simulink model "PMSM_Load_Compensation"  (R2019b)
settings: Solver=FixedStepAuto  StartTime=0.0  StopTime=4  FixedStep=2e-5  RelTol=1e-4  EnableMultiTasking=on
InitFcn:
  | Ts = 2e-5
  | Pn = 4
undefined symbols (not defined in the file or in its folder): DiscIntNeverNeededParam
libraries: dsparch4 x8, powerlib x5, simulink x2, powerlib_extras x2, powerlib_meascontrol x1
settings Model: Creator=84360  LastModifiedBy=user
settings DataIOCC: ReturnWorkspaceOutputs=off
settings OptimizationCC: LifeSpan=inf
settings DebuggingCC: SFUnexpectedBacktrackingDiag=warning  SFNoUnconditionalDefaultTransitionDiag=warning  ArithmeticOperatorsInVariantConditions=warning
settings SFSimCC: SimUseLocalCustomCode=off  CustomCodeUndefinedFunction=UseInterfaceOnly
settings RTWCC: RTWUseLocalCustomCode=off
settings CodeAppCC: StateflowObjectComments=on
settings GRTTargetCC: TargetLangStandard=C89/C90 (ANSI)  GeneratePreprocessorConditionals=Disable all
settings ConfigComp: CovMetricSettings=dw  CovHtmlReporting=on  CovSaveCumulativeToWorkspaceVar=on  CovSaveSingleToWorkspaceVar=on  CovExternalEMLEnable=off
settings SimscapeCC: SimscapeNormalizeSystem=off

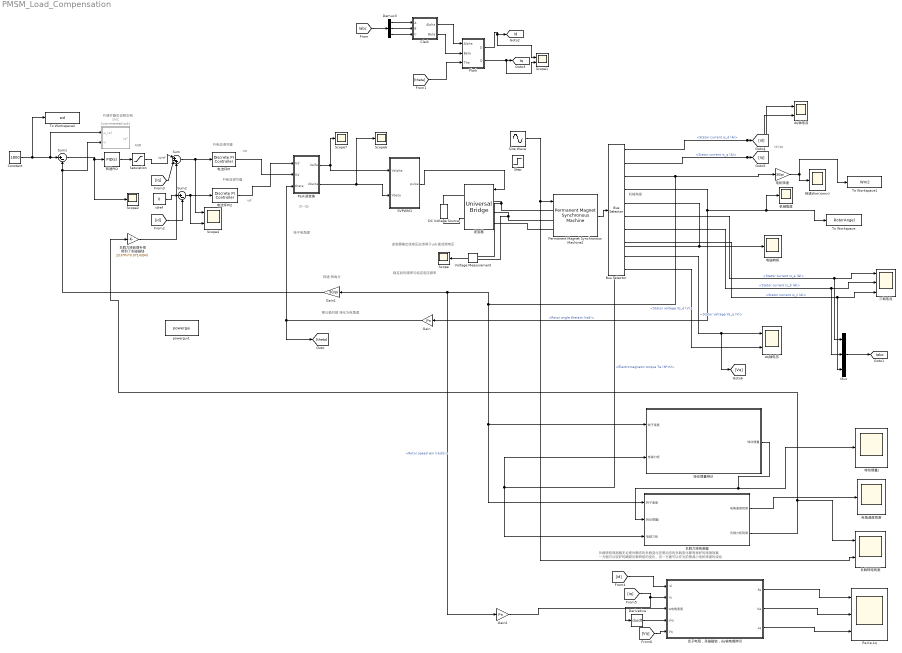
== system PMSM_Load_Compensation ==
  note: 负载转矩观测器无论是对静态的负载变化还是动态的负载变化都有很好的观测效果
      | 一方面可以较好的跟踪负载转矩的变化，另一方面可以作为前馈减小电机转速的波动
  note: PI调节器见说明文档
  note: ASR
  note: 转速 转每分
  note: 转子电角度
  note: 机械角度
  note: 2r--2s
  note: PI电流调节器
  note: ud
  note: uq
  note: iqref
  note: id,iqs
  note: PI电流调节器
  note: 乘以极对数 转化为电角度
  note: 逆变器输出线电压应该等于udc直流测电压
  note: 稳定后的频率与给定电压频率
  Bus Selector : BusSelector  OutputSignals=Stator current is_d (A),Stator current is_q (A),Rotor speed wm (rad/s),Rotor angle thetam (rad),Electromagnetic torque Te (N*m),Stator current is_a (A),Stator current is_b (A),Stator current is_c (A),Stator voltage Vs_q (V),Stator voltage Vs_d (V)
  Clark : Subsystem
  Constant : Constant  Value=1800
  DC Voltage Source : powerlib/Electrical Sources/DC Voltage Source  Amplitude=311  Measurements=None
      settings: SourceProductName=Simscape Electrical
  Demux3 : Demux  Outputs=3
  Derivative : Derivative
  Gain : Gain  Gain=Pn
  Gain1 : Gain  Gain=30/pi
  Gain2 : Gain  Gain=Pn
  Mux : Mux  Inputs=3
  Park逆变换 : Subsystem
  Permanent Magnet Synchronous Machine2 : powerlib/Machines/Permanent Magnet Synchronous Machine  NbPhases=3  FluxDistribution=Sinusoidal  RotorType=Round  MechanicalLoad=Torque Tm  PresetModel=No  ShowDetailedParameters=on  MeasurementBus=off  Resistance=0.18  Inductance=8.5e-3  dqInductances=[0.00309 0.00309]  La=0.000835  MachineConstant=Flux linkage established by magnets (V.s)  Flux=0.0714394  VoltageCst=51.8307  TorqueCst=0.42864  Flat=120  Mechanical=[0.000621417 0.000303448 4]  PolePairs=4  InitialConditions=[0,0, 0,0]  InitialConditions5ph=[0 0 0 0 0 0]  RefAngle=Aligned with phase A axis (original Park)  IterativeDiscreteModel=Trapezoidal non iterative  TsBlock=-1  TsPowergui=0
  Plark : Subsystem
  Rs,Ke,Lq : Scope  NumInputPorts=3
  SMC : Subsystem  Commented=on
  SVPWM1 : Subsystem
  Saturation : Saturate  UpperLimit=50  LowerLimit=-50
  Scope{,2,6..7} (4 alike) : Scope
  Scope1 : Scope  NumInputPorts=2
  Scope4 : Scope  NumInputPorts=2
  Sine Wave : Sin  Amplitude=15  Frequency=2  SampleTime=0
  Step : Step  Before=5  After=10  SampleTime=0
  Sum : Sum  Inputs=|+-+
  Sum1 : Sum  Inputs=|+-
  Sum2 : Sum  Inputs=|+-
  To Workspace : ToWorkspace  VariableName=RotorAngel  SaveFormat=Timeseries  SampleTime=-1
  To Workspace1 : ToWorkspace  VariableName=Wm2  SaveFormat=Timeseries  SampleTime=-1
  To Workspace2 : ToWorkspace  VariableName=wd  SaveFormat=Timeseries  SampleTime=-1
  Voltage Measurement : powerlib/Measurements/Voltage Measurement  PhasorSimulation=off  OutputType=Complex  PSBequivalent=0
      settings: SourceProductName=Simscape Electrical
  dq轴电压 : Scope  NumInputPorts=2
  dq轴电流 : Scope  NumInputPorts=2
  idref : Constant  Value=0
  powergui1 : powerlib/powergui  SimulationMode=Discrete  SampleTime=2e-5  frequency=60  Iterations=50  frequencyindice=0  Pbase=100e6  ErrMax=1e-4  UnitsV=kV  UnitsW=MW  buscounter=0  FunctionMessages=off  echomessages=off  EnableUseOfTLC=off  CurrentSourceSwitches=off  DisableSnubberDevices=off  DisableRonSwitches=off  DisableVfSwitches=off  DisplayEquations=off  AutomaticDiscreteSolvers=off  SolverType=Tustin/Backward Euler (TBE)  Interpol=off  ExternalGateDelay=off  methode=off  Ts=100  x0status=blocks  SPID=off  SwTol=0  HookPort=off  NonlinearTolerance=1e-4  nMaxIteration=100  ContinueOnMaxIteration=off  RestoreLinks=warning  ResistiveCurrentMeasurement=off  Frange=[0:2:500]  Ylog=off  Xlog=on  ShowGrid=off  save=off  variable=ZData  structure=0  ZoomFFT=on  StartTime=0.0  cycles=1  DisplayStyle=1  fundamental=60  FreqAxis=off  MaxFrequency=1000  frequencyindicesteady=1  RmsSteady=1  display=off
      settings: SourceProductName=Simscape Electrical
  三相电流 : Scope  NumInputPorts=3
  定子电阻，永磁磁链，dq轴电感辨识 : Subsystem
  机械角度 : Scope
  电机转速 : Gain  Gain=30/pi
  电流环PI : powerlib_extras/Discrete  Control Blocks/Discrete PI Controller  Kp=8.5e-3*2100  Ki=2.875*2100  Par_Limits=[250 -250]  Init=0  Ts=Ts
      settings: SourceProductName=Simscape Electrical
  电流环PI2 : powerlib_extras/Discrete  Control Blocks/Discrete PI Controller  Kp=8.5e-3*2100  Ki=2.875*2100  Par_Limits=[250 -250]  Init=0  Ts=Ts
      settings: SourceProductName=Simscape Electrical
  电磁转矩 : Scope
  电角速度观测 : Scope
  负载力矩前馈补偿 用到了永磁磁链 : Gain  Gain=2/(3*Pn*0.0714394)
  负载力矩观测器 : Subsystem
  负载转矩观测 : Scope  NumInputPorts=2
  转动惯量J : Scope
  转动惯量辨识 : Subsystem
  转速PID : simulink/Continuous/PID Controller  Controller=PID  Form=Parallel  TimeDomain=Continuous-time  SampleTime=-1  IntegratorMethod=Forward Euler  FilterMethod=Forward Euler  ControllerParametersSource=internal  P=0.476  I=2.3810  D=0  UseFilter=on  N=100  TunerSelectOption=Transfer Function Based (PID Tuner App)  InitialConditionSource=internal  InitialConditionForIntegrator=0  InitialConditionForFilter=0  DifferentiatorICPrevScaledInput=0  ExternalReset=none  TrackingMode=off  Kt=1  LimitOutput=off  UpperSaturationLimit=inf  LowerSaturationLimit=-inf  LinearizeAsGain=on  AntiWindupMode=none  Kb=1  POutMin=[]  POutMax=[]  IOutMin=[]  IOutMax=[]  DOutMin=[]  DOutMax=[]  NOutMin=[]  NOutMax=[]  SumOutMin=[]  SumOutMax=[]  SaturationOutMin=[]  SaturationOutMax=[]  PParamMin=[]  PParamMax=[]  IParamMin=[]  IParamMax=[]  DParamMin=[]  DParamMax=[]  NParamMin=[]  NParamMax=[]  KbParamMin=[]  KbParamMax=[]  KtParamMin=[]  KtParamMax=[]  KbOutMin=[]  KbOutMax=[]  KtOutMin=[]  KtOutMax=[]  IntegratorOutMin=[]  IntegratorOutMax=[]  FilterOutMin=[]  FilterOutMax=[]  SumI1OutMin=[]  SumI1OutMax=[]  SumI2OutMin=[]  SumI2OutMax=[]  SumI3OutMin=[]  SumI3OutMax=[]  SumI4OutMin=[]  SumI4OutMax=[]  SumDOutMin=[]  SumDOutMax=[]  DifferentiatorOutMin=[]  DifferentiatorOutMax=[]  FilterDiffOutCoefMin=[]  FilterDiffOutCoefMax=[]  ReciprocalOutMin=[]  ReciprocalOutMax=[]  SumDenOutMin=[]  SumDenOutMax=[]  SumNumOutMin=[]  SumNumOutMax=[]  DivideOutMin=[]  DivideOutMax=[]  IntegratorContinuousStateAttributes=''  IntegratorStateMustResolveToSignalObject=off  IntegratorRTWStateStorageClass=Auto  FilterContinuousStateAttributes=''  FilterStateMustResolveToSignalObject=off  FilterRTWStateStorageClass=Auto  ParallelPVariant=InternalParameters  IdealPVariant=Disabled  IVariant=InternalParameters  DVariant=InternalParameters  IntegratorVariant=Continuous  SatVariant=Disabled  AWVariant=Passthrough  PCopyVariant=Disabled  TRVariant=Disabled  FdbkBlocksVariant=Forward  IdealPFdbkVariant=Disabled  SatFdbkVariant=Disabled  DerivativeFilterVariant=ContFilter  NVariant=InternalParameters  NCopyVariant=Disabled  FilterICVariant=InternalICsFilter  IntegratorICVariant=InternalICs  ExternalResetVariant=Disabled  TRSumVariant=Passthrough  SumFdbkVariant=Disabled  SumVariant=Sum_PID
  转速Wm(r/min) : Scope
  逆变器 : powerlib/Power Electronics/Universal Bridge  Arms=3  SnubberResistance=1e5  SnubberCapacitance=inf  Device=IGBT / Diodes  Ron=1e-3  Lon=0  ForwardVoltages="[  0  0  ]"  ForwardVoltage=0  GTOparameters=[ 10e-6 , 20e-6 ]  IGBTparameters=[ 1e-6 , 2e-6 ]  Measurements=All voltages and currents  Measurements_2=None  converterType=Rectifier
      settings: SourceProductName=Simscape Electrical
  tag scope: Iabc=global, Id=global, Iq=global
  wires:
  Park逆变换/1(Ualfa) -> SVPWM1/1(Valpha), Scope7/1
  SVPWM1/1(pulse) -> 逆变器/1
  Voltage Measurement/1 -> Scope/1
  电流环PI/1 -> Park逆变换/2(Uq')
  Sum2/1 -> Scope4/2, 电流环PI2/1
  电流环PI2/1 -> Park逆变换/1(Ud')
  Permanent Magnet Synchronous Machine2/1 -> Bus Selector/1
  idref/1 -> Sum2/1
  Sum1/1 -> Scope2/1, 转速PID/1
  Bus Selector/4 -> To Workspace/1, 机械角度/1, Gain/1  "<Rotor angle thetam (rad)>"
  Bus Selector/3 -> 电机转速/1, Gain2/1, Gain1/1, 负载力矩观测器/1(转子速度), 转动惯量辨识/1(转子速度)  "<Rotor speed wm (rad/s)>"
  Gain/1 -> [theta], Park逆变换/3(theta)
  Bus Selector/6 -> Mux/1, 三相电流/1  "<Stator current is_a (A)>"
  Bus Selector/7 -> Mux/2, 三相电流/2  "<Stator current is_b (A)>"
  Bus Selector/8 -> Mux/3, 三相电流/3  "<Stator current is_c (A)>"
  Park逆变换/2(Ubeita) -> SVPWM1/2(Vbeta), Scope6/1
  Gain1/1 -> SMC/2(w), Sum1/2
  电机转速/1 -> To Workspace1/1, 转速Wm(r/min)/1
  Mux/1 -> [Iabc]
  [Iabc] -> Demux3/1
  Demux3/2 -> Clark/2(B)
  Plark/2(Q) -> Scope1/2, [Iq]
  Demux3/3 -> Clark/3(C)
  Clark/2(Beta) -> Plark/2(Beta)
  Demux3/1 -> Clark/1(A)
  Clark/1(Alpha) -> Plark/1(Alpha)
  [theta] -> Plark/3(The)
  Plark/1(D) -> Scope1/1, [Id]
  Saturation/1 -> Sum/1
  [iq] -> Sum/2
  [id] -> Sum2/2
  Bus Selector/9 -> [Vq], dq轴电压/1  "<Stator voltage Vs_q (V)>"
  Constant/1 -> To Workspace2/1, SMC/1(w_ref), Sum1/1
  Sum/1 -> Scope4/1, 电流环PI/1
  转速PID/1 -> Saturation/1
  Bus Selector/5 -> 电磁转矩/1, 负载力矩观测器/3(电磁力矩), 转动惯量辨识/2(电磁力矩)  "<Electromagnetic torque Te (N*m)>"
  负载力矩观测器/1(电角速度观测) -> 电角速度观测/1
  负载力矩观测器/2(负载力矩观测) -> 负载转矩观测/1, 负载力矩前馈补偿 用到了永磁磁链/1
  Sine Wave/1 -> 负载转矩观测/2, Permanent Magnet Synchronous Machine2/1
  转动惯量辨识/1(转动惯量) -> 负载力矩观测器/2(转动惯量J), 转动惯量J/1
  Bus Selector/1 -> dq轴电流/1, [id]  "<Stator current is_d (A)>"
  Bus Selector/10 -> dq轴电压/2  "<Stator voltage Vs_d (V)>"
  Bus Selector/2 -> dq轴电流/2, [iq]  "<Stator current is_q (A)>"
  负载力矩前馈补偿 用到了永磁磁链/1 -> Sum/3
  定子电阻，永磁磁链，dq轴电感辨识/1(Rs) -> Rs,Ke,Lq/1
  定子电阻，永磁磁链，dq轴电感辨识/2(Ke) -> Rs,Ke,Lq/2
  定子电阻，永磁磁链，dq轴电感辨识/3(Lq) -> Rs,Ke,Lq/3
  [id] -> 定子电阻，永磁磁链，dq轴电感辨识/1(id)
  [iq] -> Derivative/1, 定子电阻，永磁磁链，dq轴电感辨识/2(iq)
  Derivative/1 -> 定子电阻，永磁磁链，dq轴电感辨识/4(diq)
  Gain2/1 -> 定子电阻，永磁磁链，dq轴电感辨识/3(w电角速度)
  [Vq] -> 定子电阻，永磁磁链，dq轴电感辨识/5(Vq)
  connections:
  Voltage Measurement/LConn1 -- Permanent Magnet Synchronous Machine2/LConn1 -- 逆变器/LConn1
  Voltage Measurement/LConn2 -- 逆变器/LConn2 -- Permanent Magnet Synchronous Machine2/LConn2
  DC Voltage Source/RConn1 -- 逆变器/RConn1
  DC Voltage Source/LConn1 -- 逆变器/RConn2
  Permanent Magnet Synchronous Machine2/LConn3 -- 逆变器/LConn3

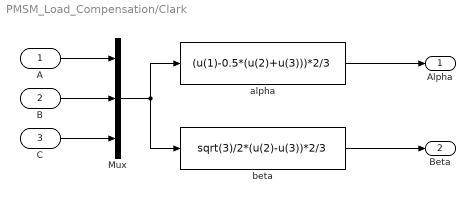
== system PMSM_Load_Compensation/Clark ==
  A : Inport
  B : Inport  Port=2
  C : Inport  Port=3
  Mux : Mux  Inputs=3
  alpha : Fcn  Expr=(u(1)-0.5*(u(2)+u(3)))*2/3
  beta : Fcn  Expr=sqrt(3)/2*(u(2)-u(3))*2/3
  Alpha : Outport
  Beta : Outport  Port=2
  wires:
  alpha/1 -> Alpha/1
  B/1 -> Mux/2
  C/1 -> Mux/3
  A/1 -> Mux/1
  Mux/1 -> beta/1, alpha/1
  beta/1 -> Beta/1

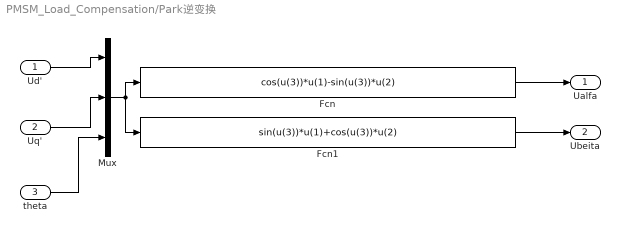
== system PMSM_Load_Compensation/Park逆变换 ==
  Ud' : Inport
  Uq' : Inport  Port=2
  theta : Inport  Port=3
  Fcn : Fcn  Expr=cos(u(3))*u(1)-sin(u(3))*u(2)
  Fcn1 : Fcn  Expr=sin(u(3))*u(1)+cos(u(3))*u(2)
  Mux : Mux  Inputs=3
  Ualfa : Outport
  Ubeita : Outport  Port=2
  wires:
  Mux/1 -> Fcn1/1, Fcn/1
  Fcn1/1 -> Ubeita/1
  Uq'/1 -> Mux/2
  Ud'/1 -> Mux/1
  Fcn/1 -> Ualfa/1
  theta/1 -> Mux/3

== system PMSM_Load_Compensation/Plark ==
  Alpha : Inport
  Beta : Inport  Port=2
  The : Inport  Port=3
  Mux : Mux  Inputs=3
  d : Fcn  Expr=u(1)*cos(u(3))+u(2)*sin(u(3))
  q : Fcn  Expr=-u(1)*sin(u(3))+u(2)*cos(u(3))
  D : Outport
  Q : Outport  Port=2
  wires:
  d/1 -> D/1
  Beta/1 -> Mux/2
  Alpha/1 -> Mux/1
  Mux/1 -> q/1, d/1
  q/1 -> Q/1
  The/1 -> Mux/3

== system PMSM_Load_Compensation/SMC ==
  w_ref : Inport
  w : Inport  Port=2
  Discrete-Time Integrator : DiscreteIntegrator  SampleTime=-1  ICPrevOutput=DiscIntNeverNeededParam  ICPrevScaledInput=DiscIntNeverNeededParam
  Mux1 : Mux  Inputs=3
  S-Function : S-Function  FunctionName=FOC_SMC  SFunctionDeploymentMode=off  EnableBusSupport=off
  Sum4 : Sum  Inputs=|+-
  iq* : Outport
  wires:
  w/1 -> Sum4/2, Mux1/2
  Sum4/1 -> Discrete-Time Integrator/1
  w_ref/1 -> Sum4/1, Mux1/1
  Discrete-Time Integrator/1 -> Mux1/3
  Mux1/1 -> S-Function/1
  S-Function/1 -> iq*/1

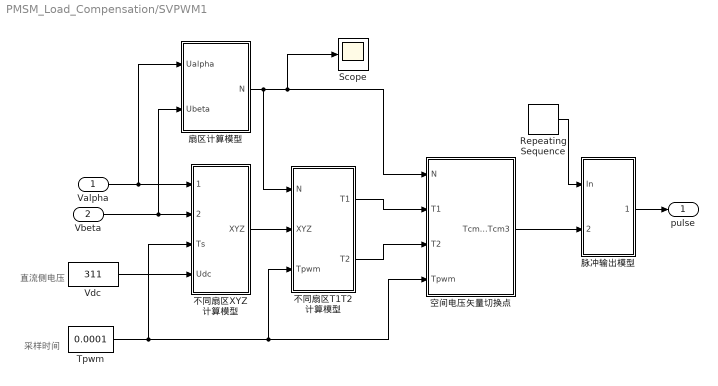
== system PMSM_Load_Compensation/SVPWM1 ==
  note: 采样时间
  note: 直流侧电压
  Valpha : Inport
  Vbeta : Inport  Port=2
  Repeating Sequence : simulink/Sources/Repeating Sequence  rep_seq_t=[0 0.00005 0.0001]  rep_seq_y=[0 0.00005 0]
  Scope : Scope
  Tpwm : Constant  Value=0.0001
  Vdc : Constant  Value=311
  不同扇区T1T2 计算模型 : Subsystem
  不同扇区XYZ 计算模型 : Subsystem
  扇区计算模型 : Subsystem
  空间电压矢量切换点 : Subsystem
  脉冲输出模型 : Subsystem
  pulse : Outport
  wires:
  脉冲输出模型/1(PWM) -> pulse/1
  Repeating Sequence/1 -> 脉冲输出模型/1(In)
  Vbeta/1 -> 不同扇区XYZ 计算模型/2(Ubeta), 扇区计算模型/2(Ubeta)
  不同扇区T1T2 计算模型/1(T1) -> 空间电压矢量切换点/2(T1)
  Valpha/1 -> 不同扇区XYZ 计算模型/1(Ualpha), 扇区计算模型/1(Ualpha)
  不同扇区T1T2 计算模型/2(T2) -> 空间电压矢量切换点/3(T2)
  扇区计算模型/1("N ") -> Scope/1, 空间电压矢量切换点/1(N), 不同扇区T1T2 计算模型/1(N)
  不同扇区XYZ 计算模型/1(XYZ) -> 不同扇区T1T2 计算模型/2(XYZ)
  Tpwm/1 -> 不同扇区XYZ 计算模型/3(Ts), 空间电压矢量切换点/4(Tpwm), 不同扇区T1T2 计算模型/3(Tpwm)
  Vdc/1 -> 不同扇区XYZ 计算模型/4(Udc)
  空间电压矢量切换点/1(Tcm1 Tcm2 Tcm3) -> 脉冲输出模型/2(Tcm123)

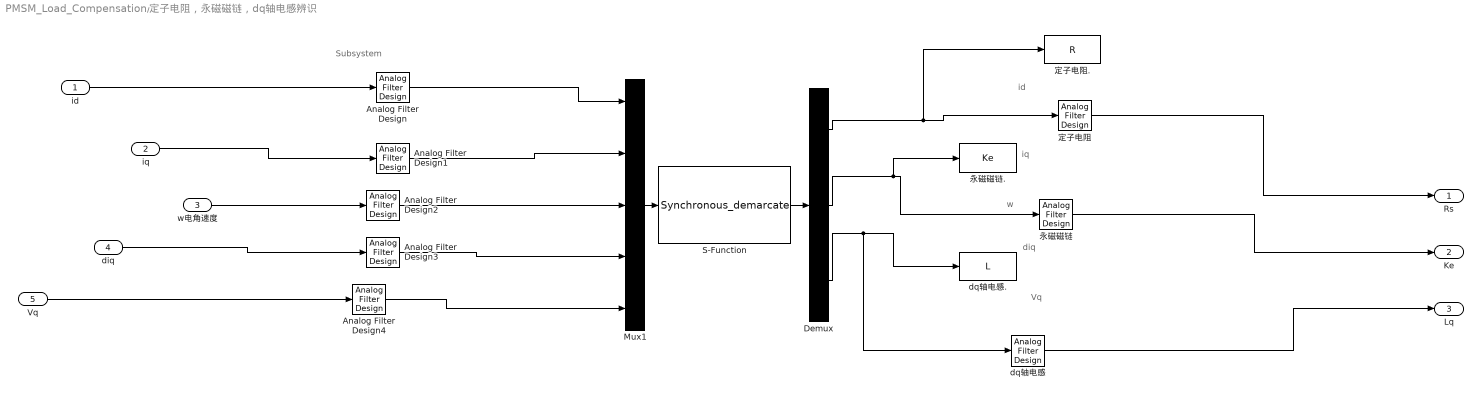
== system PMSM_Load_Compensation/定子电阻，永磁磁链，dq轴电感辨识 ==
  note: Subsystem
  note: id
  note: iq
  note: w
  note: diq
  note: Vq
  id : Inport
  iq : Inport  Port=2
  w电角速度 : Inport  Port=3
  diq : Inport  Port=4
  Vq : Inport  Port=5
  Analog Filter Design{,1..4} (5 alike) : dsparch4/Analog Filter Design  method=Butterworth  filttype=Lowpass  N=8  Wlo=50  Whi=80  Rp=2  Rs=40
  Demux : Demux  Outputs=3
  Mux1 : Mux  Inputs=5
  S-Function : S-Function  FunctionName=Synchronous_demarcate  SFunctionDeploymentMode=off  EnableBusSupport=off
  dq轴电感 : dsparch4/Analog Filter Design  method=Butterworth  filttype=Lowpass  N=8  Wlo=20  Whi=80  Rp=2  Rs=40
  dq轴电感. : ToWorkspace  VariableName=L  SaveFormat=Timeseries  SampleTime=-1
  定子电阻 : dsparch4/Analog Filter Design  method=Butterworth  filttype=Lowpass  N=8  Wlo=20  Whi=80  Rp=2  Rs=40
  定子电阻. : ToWorkspace  VariableName=R  SaveFormat=Timeseries  SampleTime=-1
  永磁磁链 : dsparch4/Analog Filter Design  method=Butterworth  filttype=Lowpass  N=8  Wlo=20  Whi=80  Rp=2  Rs=40
  永磁磁链. : ToWorkspace  VariableName=Ke  SaveFormat=Timeseries  SampleTime=-1
  Rs : Outport
  Ke : Outport  Port=2
  Lq : Outport  Port=3
  wires:
  diq/1 -> Analog Filter Design3/1
  永磁磁链/1 -> Ke/1
  iq/1 -> Analog Filter Design1/1
  定子电阻/1 -> Rs/1
  w电角速度/1 -> Analog Filter Design2/1
  S-Function/1 -> Demux/1
  id/1 -> Analog Filter Design/1
  Demux/2 -> 永磁磁链./1, 永磁磁链/1
  Analog Filter Design3/1 -> Mux1/4
  Demux/1 -> 定子电阻./1, 定子电阻/1
  Mux1/1 -> S-Function/1
  Vq/1 -> Analog Filter Design4/1
  Analog Filter Design2/1 -> Mux1/3
  dq轴电感/1 -> Lq/1
  Demux/3 -> dq轴电感./1, dq轴电感/1
  Analog Filter Design4/1 -> Mux1/5
  Analog Filter Design/1 -> Mux1/1
  Analog Filter Design1/1 -> Mux1/2

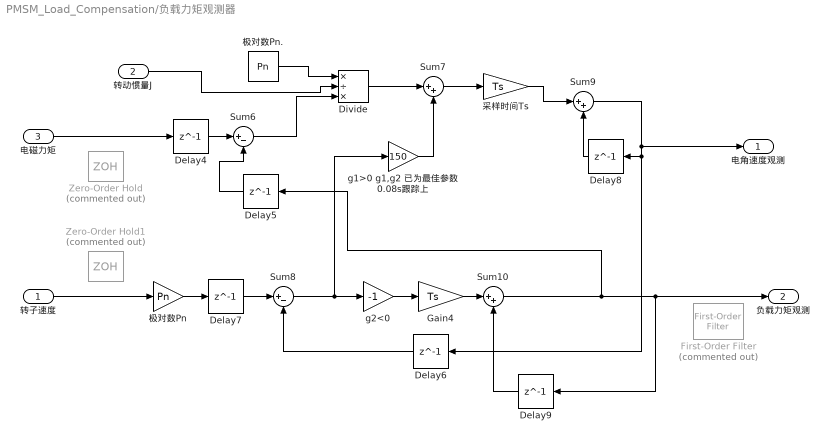
== system PMSM_Load_Compensation/负载力矩观测器 ==
  转子速度 : Inport
  转动惯量J : Inport  Port=2
  电磁力矩 : Inport  Port=3
  Delay{4..9} (6 alike) : Delay  DelayLength=1  InitialCondition=0
  Divide : Product  Inputs=*/*
  First-Order Filter : powerlib_meascontrol/Filters/First-Order Filter  Commented=on  FilterType=Lowpass  Tc=10e-3  Ts=0  Initialize=on  Vac_Init=[0, 0, 200]  Vdc_Init=0  PlotResponse=off  FreqRange="[0,  200,  1]"
      settings: SourceProductName=Simscape Electrical
  Gain4 : Gain  Gain=Ts
  Sum10 : Sum  Inputs=|++
  Sum6 : Sum  Inputs=|+-
  Sum7 : Sum  Inputs=|++
  Sum8 : Sum  Inputs=|+-
  Sum9 : Sum  Inputs=|++
  Zero-Order Hold : ZeroOrderHold  Commented=on  SampleTime=-1
  Zero-Order Hold1 : ZeroOrderHold  Commented=on  SampleTime=-1
  g1>0 g1,g2 已为最佳参数 0.08s跟踪上 : Gain  Gain=150
  g2<0 : Gain  Gain=-1
  极对数Pn : Gain  Gain=Pn
  极对数Pn. : Constant  Value=Pn
  采样时间Ts : Gain  Gain=Ts
  电角速度观测 : Outport
  负载力矩观测 : Outport  Port=2
  wires:
  Sum9/1 -> 电角速度观测/1, Delay8/1, Delay6/1
  Sum6/1 -> Divide/3
  极对数Pn/1 -> Delay7/1
  Sum7/1 -> 采样时间Ts/1
  Delay6/1 -> Sum8/2
  Delay5/1 -> Sum6/2
  g1>0 g1,g2 已为最佳参数 0.08s跟踪上/1 -> Sum7/2
  Sum8/1 -> g1>0 g1,g2 已为最佳参数 0.08s跟踪上/1, g2<0/1
  Delay7/1 -> Sum8/1
  采样时间Ts/1 -> Sum9/1
  Gain4/1 -> Sum10/1
  Delay8/1 -> Sum9/2
  Divide/1 -> Sum7/1
  g2<0/1 -> Gain4/1
  Delay9/1 -> Sum10/2
  极对数Pn./1 -> Divide/1
  Delay4/1 -> Sum6/1
  转动惯量J/1 -> Divide/2
  Sum10/1 -> Delay5/1, 负载力矩观测/1, Delay9/1
  电磁力矩/1 -> Delay4/1
  转子速度/1 -> 极对数Pn/1

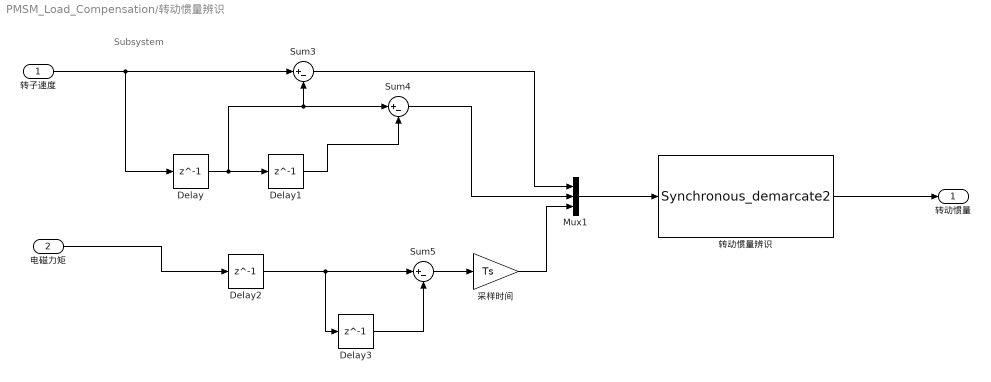
== system PMSM_Load_Compensation/转动惯量辨识 ==
  note: Subsystem
  转子速度 : Inport
  电磁力矩 : Inport  Port=2
  Delay{,1..3} (4 alike) : Delay  DelayLength=1  InitialCondition=0
  Mux1 : Mux  Inputs=3
  Sum3 : Sum  Inputs=|+-
  Sum4 : Sum  Inputs=|+-
  Sum5 : Sum  Inputs=|+-
  转动惯量辨识 : S-Function  FunctionName=Synchronous_demarcate2  SFunctionDeploymentMode=off  EnableBusSupport=off
  采样时间 : Gain  Gain=Ts
  转动惯量 : Outport
  wires:
  Mux1/1 -> 转动惯量辨识/1
  Sum5/1 -> 采样时间/1
  Delay1/1 -> Sum4/2
  采样时间/1 -> Mux1/3
  Delay/1 -> Sum3/2, Sum4/1, Delay1/1
  Sum3/1 -> Mux1/1
  Sum4/1 -> Mux1/2
  转子速度/1 -> Delay/1, Sum3/1
  Delay3/1 -> Sum5/2
  Delay2/1 -> Delay3/1, Sum5/1
  电磁力矩/1 -> Delay2/1
  转动惯量辨识/1 -> 转动惯量/1

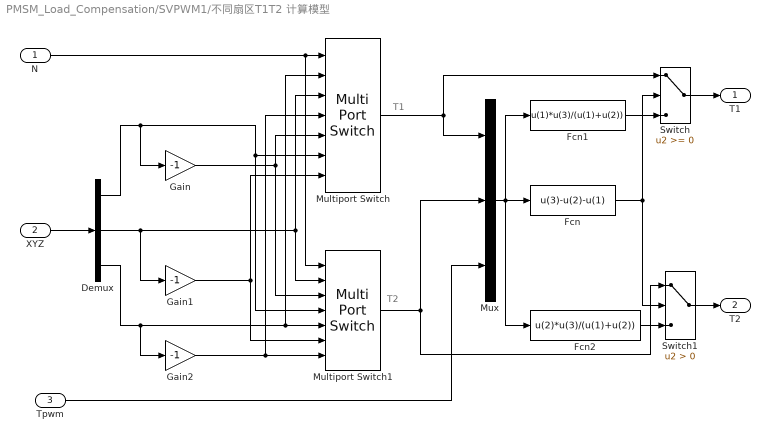
== system PMSM_Load_Compensation/SVPWM1/不同扇区T1T2 计算模型 ==
  note: T1
  note: T2
  N : Inport
  XYZ : Inport  Port=2
  Tpwm : Inport  Port=3
  Demux : Demux  Outputs=3
  Fcn : Fcn  Expr=u(3)-u(2)-u(1)
  Fcn1 : Fcn  Expr=u(1)*u(3)/(u(1)+u(2))
  Fcn2 : Fcn  Expr=u(2)*u(3)/(u(1)+u(2))
  Gain : Gain  Gain=-1
  Gain1 : Gain  Gain=-1
  Gain2 : Gain  Gain=-1
  Multiport Switch : MultiPortSwitch  Inputs=6  DiagnosticForDefault=Warning
  Multiport Switch1 : MultiPortSwitch  Inputs=6  DiagnosticForDefault=Warning
  Mux : Mux  Inputs=3
  Switch : Switch
  Switch1 : Switch  Criteria=u2 > Threshold
  T1 : Outport
  T2 : Outport  Port=2
  wires:
  Tpwm/1 -> Mux/3
  XYZ/1 -> Demux/1
  Switch1/1 -> T2/1
  Switch/1 -> T1/1
  Fcn2/1 -> Switch1/3
  Fcn1/1 -> Switch/3
  Fcn/1 -> Switch/2, Switch1/2
  Mux/1 -> Fcn1/1, Fcn/1, Fcn2/1
  Multiport Switch/1 -> Switch/1, Mux/1
  Multiport Switch1/1 -> Switch1/1, Mux/2
  N/1 -> Multiport Switch/1, Multiport Switch1/1
  Demux/2 -> Multiport Switch/3, Multiport Switch1/2, Gain1/1
  Demux/3 -> Multiport Switch1/5, Multiport Switch/2, Gain2/1
  Demux/1 -> Multiport Switch/6, Multiport Switch1/4, Gain/1
  Gain/1 -> Multiport Switch1/3, Multiport Switch/5
  Gain2/1 -> Multiport Switch/4, Multiport Switch1/7
  Gain1/1 -> Multiport Switch1/6, Multiport Switch/7

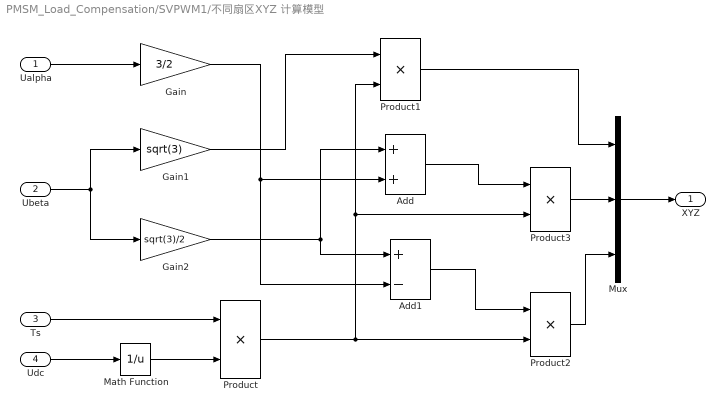
== system PMSM_Load_Compensation/SVPWM1/不同扇区XYZ 计算模型 ==
  Ualpha : Inport
  Ubeta : Inport  Port=2
  Ts : Inport  Port=3
  Udc : Inport  Port=4
  Add : Sum
  Add1 : Sum  Inputs=+-
  Gain : Gain  Gain=3/2
  Gain1 : Gain  Gain=sqrt(3)
  Gain2 : Gain  Gain=sqrt(3)/2
  Math Function : Math  Operator=reciprocal  SaturateOnIntegerOverflow=on
  Mux : Mux  Inputs=3
  Product{,1..3} (4 alike) : Product  RndMeth=Zero
  XYZ : Outport
  wires:
  Mux/1 -> XYZ/1
  Product1/1 -> Mux/1
  Product3/1 -> Mux/2
  Product2/1 -> Mux/3
  Ualpha/1 -> Gain/1
  Ubeta/1 -> Gain2/1, Gain1/1
  Udc/1 -> Math Function/1
  Math Function/1 -> Product/2
  Ts/1 -> Product/1
  Gain1/1 -> Product1/1
  Product/1 -> Product2/2, Product1/2, Product3/2
  Gain/1 -> Add1/2, Add/2
  Gain2/1 -> Add/1, Add1/1
  Add1/1 -> Product2/1
  Add/1 -> Product3/1

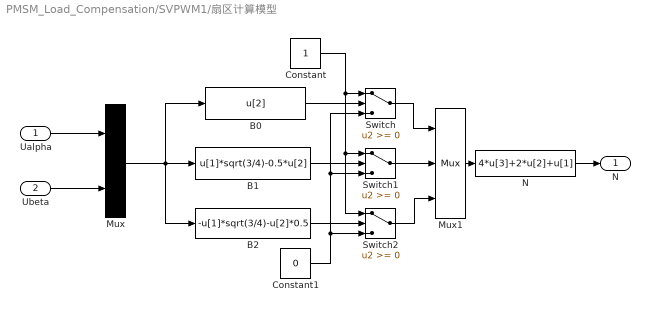
== system PMSM_Load_Compensation/SVPWM1/扇区计算模型 ==
  Ualpha : Inport
  Ubeta : Inport  Port=2
  B0 : Fcn  Expr=u[2]
  B1 : Fcn  Expr=u[1]*sqrt(3/4)-0.5*u[2]
  B2 : Fcn  Expr=-u[1]*sqrt(3/4)-u[2]*0.5
  Constant : Constant
  Constant1 : Constant  Value=0
  Mux : Mux  Inputs=2
  Mux1 : Mux  Inputs=3
  N : Fcn  Expr=4*u[3]+2*u[2]+u[1]
  Switch : Switch
  Switch1 : Switch
  Switch2 : Switch
  "N " : Outport
  wires:
  Switch2/1 -> Mux1/3
  Switch/1 -> Mux1/1
  Ualpha/1 -> Mux/1
  Ubeta/1 -> Mux/2
  Mux/1 -> B2/1, B1/1, B0/1
  B0/1 -> Switch/2
  B1/1 -> Switch1/2
  B2/1 -> Switch2/2
  Constant/1 -> Switch/1, Switch2/1, Switch1/1
  Constant1/1 -> Switch/3, Switch1/3, Switch2/3
  Switch1/1 -> Mux1/2
  Mux1/1 -> N/1
  N/1 -> "N "/1

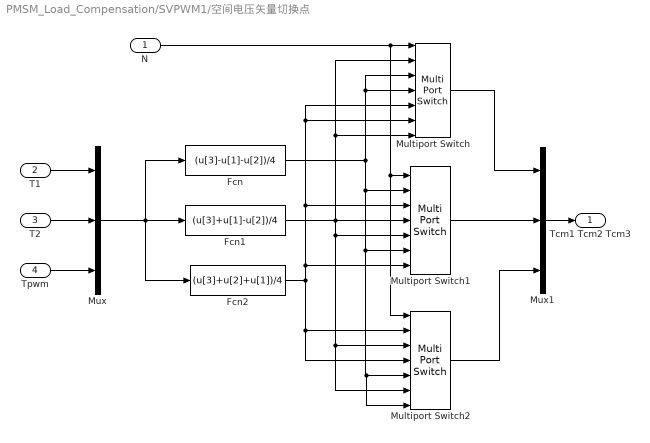
== system PMSM_Load_Compensation/SVPWM1/空间电压矢量切换点 ==
  N : Inport
  T1 : Inport  Port=2
  T2 : Inport  Port=3
  Tpwm : Inport  Port=4
  Fcn : Fcn  Expr=(u[3]-u[1]-u[2])/4
  Fcn1 : Fcn  Expr=(u[3]+u[1]-u[2])/4
  Fcn2 : Fcn  Expr=(u[3]+u[2]+u[1])/4
  Multiport Switch : MultiPortSwitch  Inputs=6  DiagnosticForDefault=Warning
  Multiport Switch1 : MultiPortSwitch  Inputs=6  DiagnosticForDefault=Warning
  Multiport Switch2 : MultiPortSwitch  Inputs=6  DiagnosticForDefault=Warning
  Mux : Mux  Inputs=3
  Mux1 : Mux  Inputs=3
  Tcm1 Tcm2 Tcm3 : Outport
  wires:
  Mux/1 -> Fcn2/1, Fcn/1, Fcn1/1
  Tpwm/1 -> Mux/3
  T2/1 -> Mux/2
  T1/1 -> Mux/1
  Multiport Switch2/1 -> Mux1/3
  Multiport Switch1/1 -> Mux1/2
  Multiport Switch/1 -> Mux1/1
  Mux1/1 -> Tcm1 Tcm2 Tcm3/1
  Fcn/1 -> Multiport Switch/3, Multiport Switch/4, Multiport Switch1/6, Multiport Switch2/5, Multiport Switch2/7, Multiport Switch1/2
  Fcn1/1 -> Multiport Switch1/5, Multiport Switch2/3, Multiport Switch2/6, Multiport Switch1/4, Multiport Switch/7, Multiport Switch/2
  Fcn2/1 -> Multiport Switch/5, Multiport Switch/6, Multiport Switch1/3, Multiport Switch1/7, Multiport Switch2/2, Multiport Switch2/4
  N/1 -> Multiport Switch2/1, Multiport Switch1/1, Multiport Switch/1

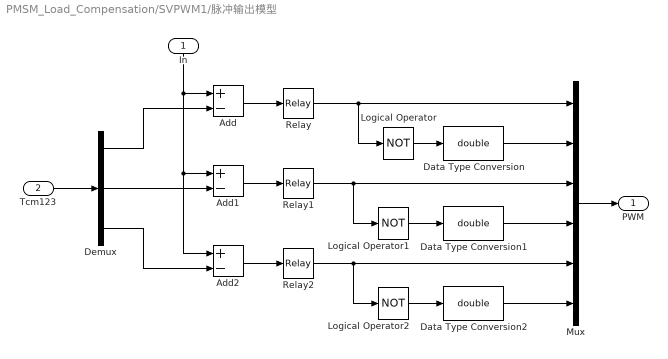
== system PMSM_Load_Compensation/SVPWM1/脉冲输出模型 ==
  In : Inport
  Tcm123 : Inport  Port=2
  Add : Sum  Inputs=+-
  Add1 : Sum  Inputs=+-
  Add2 : Sum  Inputs=+-
  Data Type Conversion : DataTypeConversion  OutDataTypeStr=double
  Data Type Conversion1 : DataTypeConversion  OutDataTypeStr=double
  Data Type Conversion2 : DataTypeConversion  OutDataTypeStr=double
  Demux : Demux  Outputs=3
  Logical Operator : Logic  Operator=NOT  AllPortsSameDT=off  OutDataTypeStr=boolean
  Logical Operator1 : Logic  Operator=NOT  AllPortsSameDT=off  OutDataTypeStr=boolean
  Logical Operator2 : Logic  Operator=NOT  AllPortsSameDT=off  OutDataTypeStr=boolean
  Mux : Mux  Inputs=6
  Relay : Relay  OffSwitchValue=-eps
  Relay1 : Relay  OffSwitchValue=-eps
  Relay2 : Relay  OffSwitchValue=-eps
  PWM : Outport
  wires:
  Demux/3 -> Add2/2
  Demux/2 -> Add1/2
  Demux/1 -> Add/2
  Relay2/1 -> Mux/5, Logical Operator2/1
  Relay1/1 -> Mux/3, Logical Operator1/1
  Relay/1 -> Logical Operator/1, Mux/1
  Mux/1 -> PWM/1
  Data Type Conversion/1 -> Mux/2
  Data Type Conversion1/1 -> Mux/4
  Data Type Conversion2/1 -> Mux/6
  Logical Operator2/1 -> Data Type Conversion2/1
  Logical Operator1/1 -> Data Type Conversion1/1
  Logical Operator/1 -> Data Type Conversion/1
  Add1/1 -> Relay1/1
  Add2/1 -> Relay2/1
  Add/1 -> Relay/1
  In/1 -> Add/1, Add2/1, Add1/1
  Tcm123/1 -> Demux/1
